simulink model "ROS_01"  (R2022b)
settings: Solver=FixedStepAuto  StartTime=0.0  StopTime=inf  RelTol=1e-3
model workspace (MAT data in the model file):
  SL_ROS_VariableLengthArrays_MaxSizes.CommonInfo.ArrayTruncateAction = 'EmitWarning'
  SL_ROS_VariableLengthArrays_MaxSizes.MsgTypeMap = containers.Map
  SL_ROS_VariableLengthArrays_MaxSizes.MsgTypeMap.serialization.keys = {'sensor_msgs/CompressedImage', 'sensor_msgs/LaserScan', 'std_msgs/Int8MultiArray'}
  SL_ROS_VariableLengthArrays_MaxSizes.MsgTypeMap.serialization.values{1}(1).PropertyName = 'Data'
  SL_ROS_VariableLengthArrays_MaxSizes.MsgTypeMap.serialization.values{1}(1).DataType = 'uint8'
  SL_ROS_VariableLengthArrays_MaxSizes.MsgTypeMap.serialization.values{1}(1).MaxLength = 83420
  SL_ROS_VariableLengthArrays_MaxSizes.MsgTypeMap.serialization.values{1}(2).PropertyName = 'Format'
  SL_ROS_VariableLengthArrays_MaxSizes.MsgTypeMap.serialization.values{1}(2).DataType = 'uint8'
  SL_ROS_VariableLengthArrays_MaxSizes.MsgTypeMap.serialization.values{1}(2).MaxLength = 8
  SL_ROS_VariableLengthArrays_MaxSizes.MsgTypeMap.serialization.values{2}(1).PropertyName = 'Intensities'
  SL_ROS_VariableLengthArrays_MaxSizes.MsgTypeMap.serialization.values{2}(1).DataType = 'single'
  SL_ROS_VariableLengthArrays_MaxSizes.MsgTypeMap.serialization.values{2}(1).MaxLength = 128
  SL_ROS_VariableLengthArrays_MaxSizes.MsgTypeMap.serialization.values{2}(2).PropertyName = 'Ranges'
  SL_ROS_VariableLengthArrays_MaxSizes.MsgTypeMap.serialization.values{2}(2).DataType = 'single'
  SL_ROS_VariableLengthArrays_MaxSizes.MsgTypeMap.serialization.values{2}(2).MaxLength = 360
  SL_ROS_VariableLengthArrays_MaxSizes.MsgTypeMap.serialization.values{3}.PropertyName = 'Data'
  SL_ROS_VariableLengthArrays_MaxSizes.MsgTypeMap.serialization.values{3}.DataType = 'int8'
  SL_ROS_VariableLengthArrays_MaxSizes.MsgTypeMap.serialization.values{3}.MaxLength = 2
  SL_ROS_VariableLengthArrays_MaxSizes.MsgTypeMap.serialization.uniformity = 0
  SL_ROS_VariableLengthArrays_MaxSizes.MsgTypeMap.serialization.keyType = 'char'
  SL_ROS_VariableLengthArrays_MaxSizes.MsgTypeMap.serialization.valueType = 'any'
undefined symbols (not defined in the file): Data, Data_SL_Info
libraries: robotlib x6
settings Model: Creator=Musta  LastModifiedBy=mustacchim
settings OptimizationCC: EnhancedBackFolding=on  PassReuseOutputArgsAs=Individual arguments  ZeroExternalMemoryAtStartup=off  ZeroInternalMemoryAtStartup=off  MaxStackSize=64  OptimizeBlockOrder=speed  DifferentSizesBufferReuse=on  OptimizationCustomize=off  EfficientTunableParamExpr=on
settings DebuggingCC: ParameterTunabilityLossMsg=error
settings HardwareCC: ProdBitPerPointer=32  ProdBitPerSizeT=32  ProdBitPerPtrDiffT=32  ProdLargestAtomicFloat=None  ProdIntDivRoundTo=Undefined  ProdEndianess=Unspecified  ProdWordSize=32  ProdHWDeviceType=Generic->Unspecified (assume 32-bit Generic)
settings SFSimCC: MATLABDynamicMemAlloc=off
settings RTWCC: Description=Embedded Coder  SystemTargetFile=ert.tlc  HardwareBoard=Robot Operating System (ROS)  TLCOptions="-aInlineSetEventsForThisBaseRateFcn=TLC_FALSE -aSuppressMultiTaskScheduler=TLC_FALSE  -aRateBasedStepFcn=0"  TemplateMakefile=ert_default_tmf  Toolchain=Catkin  TargetLang=C++
settings CodeAppCC: ForceParamTrailComments=on  IgnoreCustomStorageClasses=off  OperatorAnnotations=on  SimulinkDataObjDesc=on  SFDataObjDesc=on  InsertBlockDesc=on

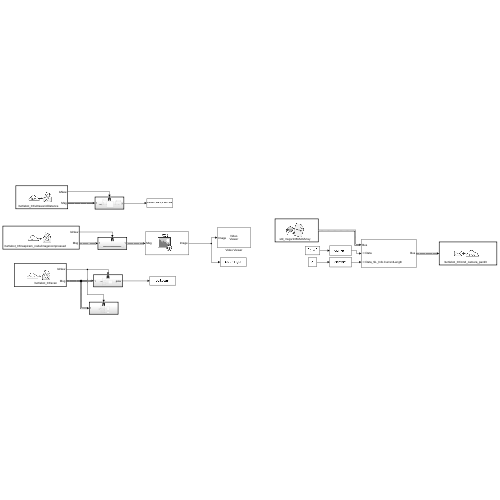
[thumbnail: Simulink's stored preview of the top-level diagram]
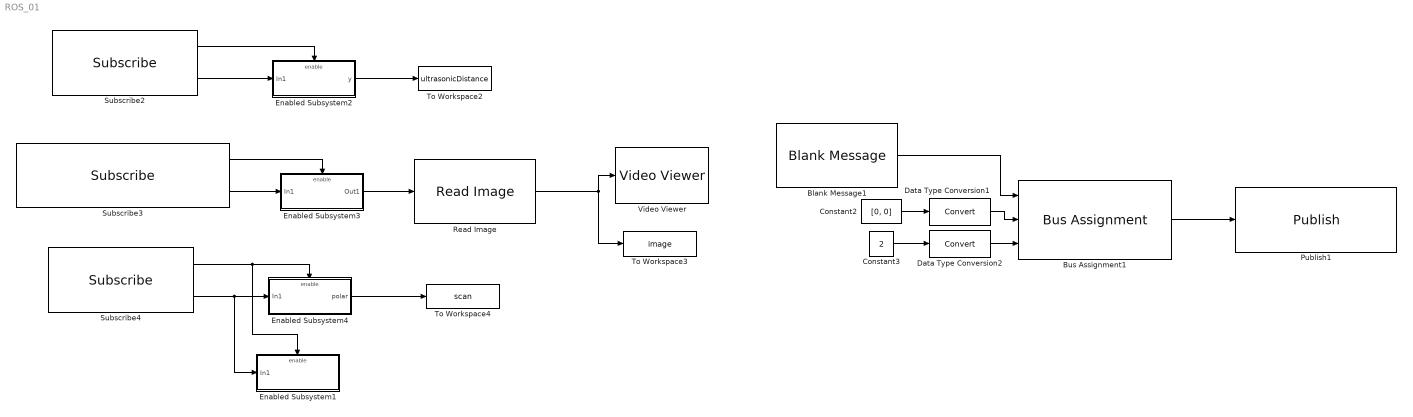
== system ROS_01 ==
  Blank Message1 : robotlib/Blank Message  messageClass=Message  entityType=std_msgs/Int8MultiArray  messageType=std_msgs/Int8MultiArray  SampleTime=-1  legacyBusStruct=off
      settings: LibrarySourceBlock=roslib/ROS/Blank Message
  Bus Assignment1 : BusAssignment  AssignedSignals=Data,Data_SL_Info.CurrentLength
  Constant2 : Constant  Value=[0, 0]
  Constant3 : Constant  Value=2
  Data Type Conversion1 : DataTypeConversion  SaturateOnIntegerOverflow=off  RndMeth=Floor
  Data Type Conversion2 : DataTypeConversion  SaturateOnIntegerOverflow=off  RndMeth=Floor
  Enabled Subsystem1 : Subsystem  TreatAsAtomicUnit=on
  Enabled Subsystem2 : Subsystem  TreatAsAtomicUnit=on
  Enabled Subsystem3 : Subsystem  TreatAsAtomicUnit=on
  Enabled Subsystem4 : Subsystem  TreatAsAtomicUnit=on
  Publish1 : robotlib/Publish  topicSource=Select from ROS network  topic=/turtlebot_03/cmd_camera_pantilt  messageType=std_msgs/Int8MultiArray  legacyBusStruct=off  messageQueueLength=1
      settings: LibrarySourceBlock=roslib/ROS/Publish
  Read Image : robotlib/Read Image  MaximumImageSize=[308, 410]  ImageEncoding=bgr8  ShowAlphaOutput=off  ShowErrorCodeOutput=off  VariableSizeOutputs=off
      settings: LibrarySourceBlock=roslib/ROS/Read Image
  Subscribe2 : robotlib/Subscribe  topicSource=Select from ROS network  topic=/turtlebot_03/ultrasonicDistance  messageType=std_msgs/Float32  SampleTime=0.11  legacyBusStruct=off  messageQueueLength=1
      settings: LibrarySourceBlock=roslib/ROS/Subscribe
  Subscribe3 : robotlib/Subscribe  topicSource=Select from ROS network  topic=/turtlebot_03/raspicam_node/image/compressed  messageType=sensor_msgs/CompressedImage  SampleTime=0.03  legacyBusStruct=off  messageQueueLength=1
      settings: LibrarySourceBlock=roslib/ROS/Subscribe
  Subscribe4 : robotlib/Subscribe  topicSource=Select from ROS network  topic=/turtlebot_03/scan  messageType=sensor_msgs/LaserScan  SampleTime=0.16  legacyBusStruct=off  messageQueueLength=1
      settings: LibrarySourceBlock=roslib/ROS/Subscribe
  To Workspace2 : ToWorkspace  VariableName=ultrasonicDistance  SaveFormat=Structure With Time  SampleTime=-1
  To Workspace3 : ToWorkspace  VariableName=image  SaveFormat=Structure With Time  SampleTime=-1
  To Workspace4 : ToWorkspace  VariableName=scan  SaveFormat=Structure With Time  SampleTime=-1
  Video Viewer : VideoViewer  FigPos=[832 638 418 317]
  wires:
  Subscribe4/1 -> Enabled Subsystem1/Enable, Enabled Subsystem4/Enable
  Enabled Subsystem3/1(Out1) -> Read Image/1
  Subscribe3/2 -> Enabled Subsystem3/1(In1)
  Subscribe4/2 -> Enabled Subsystem1/1(In1), Enabled Subsystem4/1(In1)
  Subscribe3/1 -> Enabled Subsystem3/Enable
  Subscribe2/2 -> Enabled Subsystem2/1(In1)
  Enabled Subsystem2/1(y) -> To Workspace2/1
  Enabled Subsystem4/1(polar) -> To Workspace4/1
  Subscribe2/1 -> Enabled Subsystem2/Enable
  Read Image/1 -> Video Viewer/1, To Workspace3/1
  Constant3/1 -> Data Type Conversion2/1
  Constant2/1 -> Data Type Conversion1/1
  Data Type Conversion2/1 -> Bus Assignment1/3
  Data Type Conversion1/1 -> Bus Assignment1/2
  Blank Message1/1 -> Bus Assignment1/1
  Bus Assignment1/1 -> Publish1/1

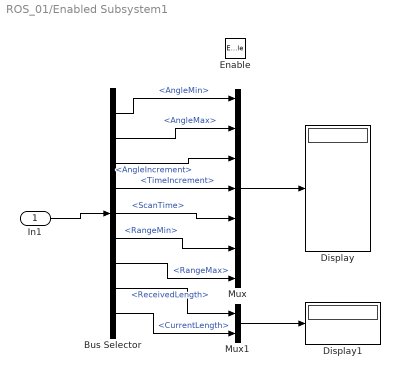
== system ROS_01/Enabled Subsystem1 ==
  In1 : Inport
  Enable : EnablePort
  Bus Selector : BusSelector  OutputSignals=AngleMin,AngleMax,AngleIncrement,TimeIncrement,ScanTime,RangeMin,RangeMax,Ranges_SL_Info.ReceivedLength,Ranges_SL_Info.CurrentLength
  Display : Display
  Display1 : Display
  Mux : Mux  Inputs=7
  Mux1 : Mux  Inputs=2
  wires:
  In1/1 -> Bus Selector/1
  Mux/1 -> Display/1
  Bus Selector/1 -> Mux/1  "<AngleMin>"
  Bus Selector/2 -> Mux/2  "<AngleMax>"
  Bus Selector/3 -> Mux/3  "<AngleIncrement>"
  Bus Selector/4 -> Mux/4  "<TimeIncrement>"
  Bus Selector/5 -> Mux/5  "<ScanTime>"
  Bus Selector/6 -> Mux/6  "<RangeMin>"
  Bus Selector/7 -> Mux/7  "<RangeMax>"
  Bus Selector/8 -> Mux1/1  "<ReceivedLength>"
  Bus Selector/9 -> Mux1/2  "<CurrentLength>"
  Mux1/1 -> Display1/1

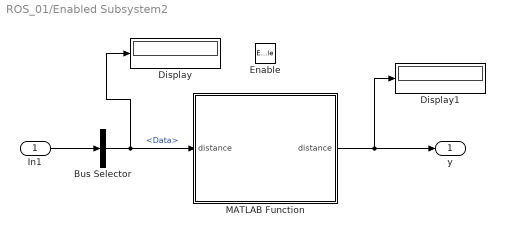
== system ROS_01/Enabled Subsystem2 ==
  In1 : Inport
  Enable : EnablePort
  Bus Selector : BusSelector  OutputSignals=Data
  Display : Display
  Display1 : Display
  MATLAB Function : MATLAB Function  TreatAsAtomicUnit=on
  y : Outport
  wires:
  In1/1 -> Bus Selector/1
  Bus Selector/1 -> Display/1, MATLAB Function/1("distance ")  "<Data>"
  MATLAB Function/1(distance) -> Display1/1, y/1

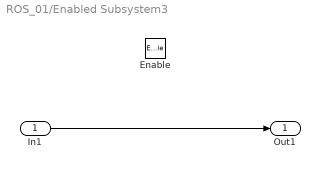
== system ROS_01/Enabled Subsystem3 ==
  In1 : Inport
  Enable : EnablePort
  Out1 : Outport
  wires:
  In1/1 -> Out1/1

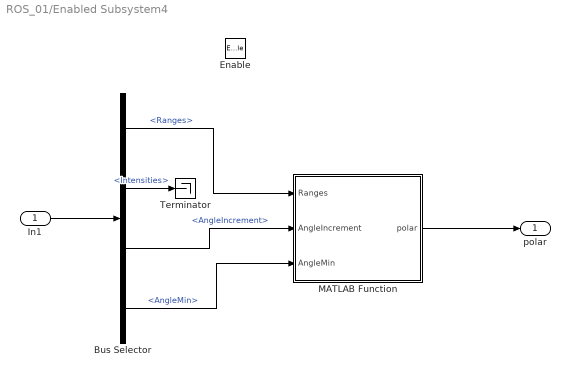
== system ROS_01/Enabled Subsystem4 ==
  In1 : Inport
  Enable : EnablePort
  Bus Selector : BusSelector  OutputSignals=Ranges,Intensities,AngleIncrement,AngleMin
  MATLAB Function : MATLAB Function  TreatAsAtomicUnit=on
  Terminator : Terminator
  polar : Outport
  wires:
  Bus Selector/1 -> MATLAB Function/1(Ranges)  "<Ranges>"
  In1/1 -> Bus Selector/1
  Bus Selector/4 -> MATLAB Function/3(AngleMin)  "<AngleMin>"
  Bus Selector/3 -> MATLAB Function/2(AngleIncrement)  "<AngleIncrement>"
  Bus Selector/2 -> Terminator/1  "<Intensities>"
  MATLAB Function/1(polar) -> polar/1

== matlab function ROS_01/Enabled Subsystem4/MATLAB Function ==
  data: Ranges input; polar output; AngleIncrement input; AngleMin input
function polar = fcn(Ranges, AngleIncrement, AngleMin)

    polar = zeros(length(Ranges), 2);
    for i = 1:length(Ranges)
        polar(i,1) = Ranges(i);
        polar(i,2) = AngleMin + ((i-1) * AngleIncrement);
    end

end

== matlab function ROS_01/Enabled Subsystem2/MATLAB Function ==
  data: distance input; distance output
function distance = discard_ultrasonic(distance)

%     % if out of ranges -> discard
%     x = randn(10,1);
%     indices = find(abs(x)>4.5);
%     x(indices) = [];

    % if invalid measure -> assign a flag measure not to be trusted
    indices = find(abs(distance)>4.5);
    distance(indices) = NaN;

end
